simulink model "EnrouleurHG"  (R2024b)
settings: Solver=VariableStepAuto  StartTime=0.0  StopTime=.8  RelTol=1e-3
InitFcn:
  | run("parametres.m");
values from neighbouring files (symbols this model uses):
  fv = 0    [parametres.m]
  ISAT = 4    [parametres.m]
  Jm = 13.1/1000/10000    (= 1.31e-06)    [parametres.m]
  Kadapt = Kcapt/Rt    (= 52.1518917524)    [parametres.m]
  Kcapt = 8192/2/pi    (= 1303.79729381)    [parametres.m]
  Kcm = 25.5e-3    (= 0.0255)    [parametres.m]
  KCou_I = 900    [parametres.m]
  KCou_P = 2000    [parametres.m]
  KDSI = KPos_D*80/1000000    (= 0.0736)    [parametres.m]
  Kem = 1/(374 *2*pi/60)    (= 0.0255328785709)    [parametres.m]
  KPos_I = 270    [parametres.m]
  KPos_P = 215    [parametres.m]
  KPSI = KPos_P*10/1000    (= 2.15)    [parametres.m]
  Lm = 0.77e-3    (= 0.00077)    [parametres.m]
  r = 1/18    (= 0.0555555555556)    [parametres.m]
  Rm = 7.36    [parametres.m]
  Rt = 25    [parametres.m]
  Unom = 24    [parametres.m]
libraries: simulink x2
settings Model: Creator=xavier.pessoles2  LastModifiedBy=xpess

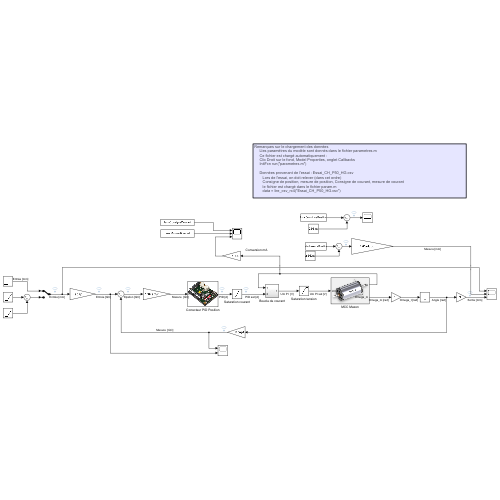
[thumbnail: Simulink's stored preview of the top-level diagram]
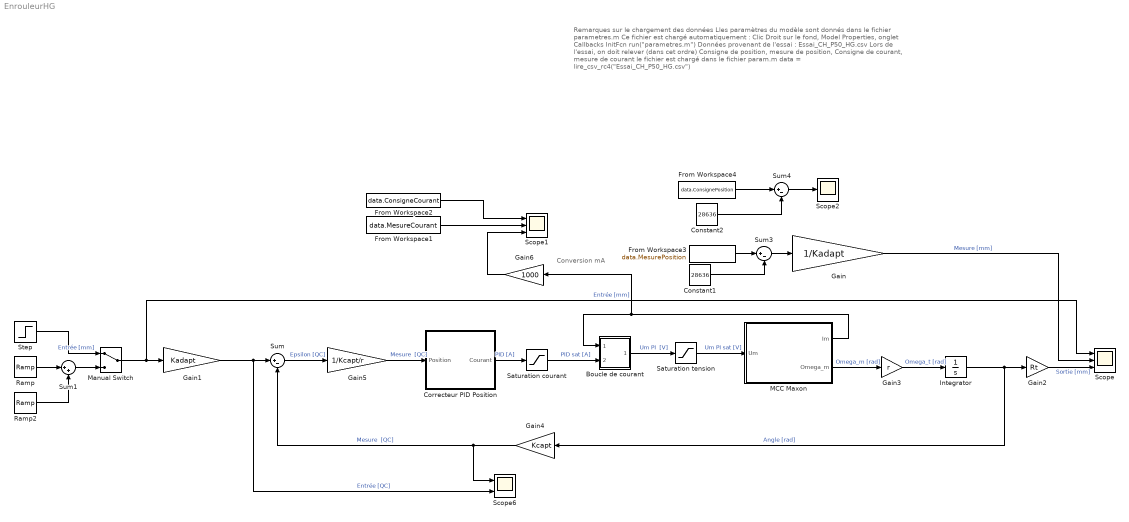
== system EnrouleurHG ==
  note: Conversion mA
  note: Remarques sur le chargement des données
      |      Lles paramètres du modèle sont donnés dans le fichier parametres.m
      |      Ce fichier est chargé automatiquement :
      |      Clic Droit sur le fond, Model Properties, onglet Callbacks
      |      InitFcn run("parametres.m")
      |
      |      Données provenant de l'essai : Essai_CH_P50_HG.csv
      |         Lors de l'essai, on doit relever (dans cet ordre)
      |         Consigne de position, mesure de position, Consigne de courant, mesure de courant
      |         le fichier est chargé dans le fichier param.m
      |         data = lire_csv_rc4("Essai_CH_P50_HG.csv")
  Boucle de courant : Subsystem
  Constant1 : Constant  Value=28636
  Constant2 : Constant  Value=28636
  Correcteur PID Position : Subsystem
      mask Display: image('EPOS.png');
  From Workspace1 : FromWorkspace  VariableName=data.MesureCourant  SampleTime=0.01
  From Workspace2 : FromWorkspace  VariableName=data.ConsigneCourant  SampleTime=0.01
  From Workspace3 : FromWorkspace  VariableName=data.MesurePosition  SampleTime=0.01
  From Workspace4 : FromWorkspace  VariableName=data.ConsignePosition  SampleTime=0.01
  Gain : Gain  Gain=1/Kadapt
  Gain1 : Gain  Gain=Kadapt
  Gain2 : Gain  Gain=Rt
  Gain3 : Gain  Gain=r
  Gain4 : Gain  Gain=Kcapt
  Gain5 : Gain  Gain=1/Kcapt/r
  Gain6 : Gain  Gain=1000
  Integrator : Integrator
  MCC Maxon : Subsystem
      mask Display: image('MCC.png');
  Manual Switch : ManualSwitch
  Ramp : simulink/Sources/Ramp  slope=378  start=0  InitialOutput=0
  Ramp2 : simulink/Sources/Ramp  slope=-378  start=1  InitialOutput=0
  Saturation courant : Saturate  UpperLimit=ISAT  LowerLimit=-ISAT
  Saturation tension : Saturate  UpperLimit=Unom  LowerLimit=-Unom
  Scope : Scope  NumInputPorts=3
  Scope1 : Scope  NumInputPorts=3
  Scope2 : Scope
  Scope6 : Scope  NumInputPorts=2
  Step : Step  Time=.08  After=50  SampleTime=0
  Sum : Sum  Inputs=|+-
  Sum1 : Sum  Inputs=|++
  Sum3 : Sum  Inputs=|+-
  Sum4 : Sum  Inputs=|+-
  wires:
  Gain3/1 -> Integrator/1  "Omega_t [rad]"
  MCC Maxon/2(Omega_m) -> Gain3/1  "Omega_m [rad]"
  Sum/1 -> Gain5/1  "Epsilon [QC]"
  MCC Maxon/1(Im) -> Gain6/1, Boucle de courant/1(In1)
  Correcteur PID Position/1(Courant) -> Saturation courant/1  "PID [A]"
  Boucle de courant/1(Out1) -> Saturation tension/1  "Um PI  [V]"
  Gain4/1 -> Scope6/1, Sum/2  "Mesure  [QC]"
  Gain1/1 -> Sum/1, Scope6/2  "Entrée [QC]"
  Gain2/1 -> Scope/3  "Sortie [mm]"
  Saturation tension/1 -> MCC Maxon/1(Um)  "Um PI sat [V]"
  Saturation courant/1 -> Boucle de courant/2(In2)  "PID sat [A]"
  Integrator/1 -> Gain2/1, Gain4/1  "Angle [rad]"
  Ramp/1 -> Sum1/1
  Ramp2/1 -> Sum1/2
  Sum1/1 -> Manual Switch/2
  Manual Switch/1 -> Gain1/1, Scope/1  "Entrée [mm]"
  Gain5/1 -> Correcteur PID Position/1(Position)  "Mesure  [QC]"
  Step/1 -> Manual Switch/1  "Entrée [mm]"
  From Workspace1/1 -> Scope1/2
  From Workspace2/1 -> Scope1/1
  From Workspace4/1 -> Sum4/1
  Gain/1 -> Scope/2  "Mesure [mm]"
  From Workspace3/1 -> Sum3/1
  Sum3/1 -> Gain/1
  Constant1/1 -> Sum3/2
  Constant2/1 -> Sum4/2
  Sum4/1 -> Scope2/1
  Gain6/1 -> Scope1/3

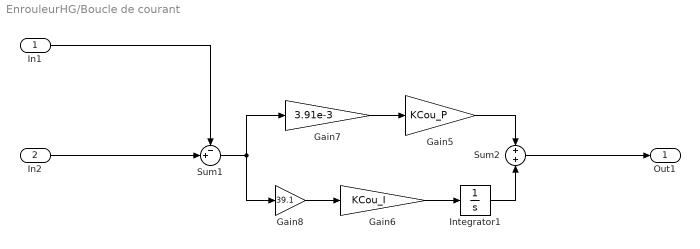
== system EnrouleurHG/Boucle de courant ==
  In1 : Inport
  In2 : Inport  Port=2
  Gain5 : Gain  Gain=KCou_P
  Gain6 : Gain  Gain=KCou_I
  Gain7 : Gain  Gain=3.91e-3
  Gain8 : Gain  Gain=39.1
  Integrator1 : Integrator
  Sum1 : Sum  Inputs=-+|
  Sum2 : Sum  Inputs=+|+
  Out1 : Outport
  wires:
  Sum1/1 -> Gain7/1, Gain8/1
  Gain5/1 -> Sum2/1
  Sum2/1 -> Out1/1
  Integrator1/1 -> Sum2/2
  Gain8/1 -> Gain6/1
  In1/1 -> Sum1/1
  Gain7/1 -> Gain5/1
  Gain6/1 -> Integrator1/1
  In2/1 -> Sum1/2

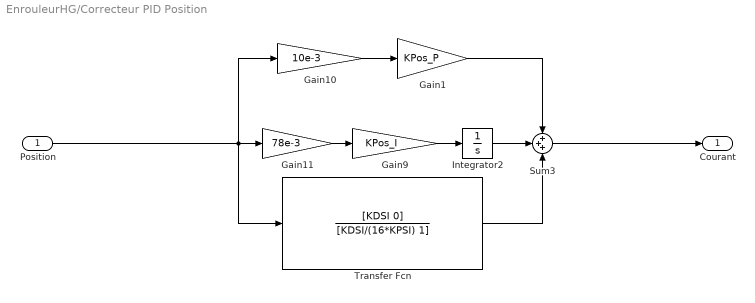
== system EnrouleurHG/Correcteur PID Position ==
  Position : Inport
  Gain1 : Gain  Gain=KPos_P
  Gain10 : Gain  Gain=10e-3
  Gain11 : Gain  Gain=78e-3
  Gain9 : Gain  Gain=KPos_I
  Integrator2 : Integrator
  Sum3 : Sum  Inputs=+++
  Transfer Fcn : TransferFcn  Numerator=[KDSI 0]  Denominator=[KDSI/(16*KPSI) 1]
  Courant : Outport
  wires:
  Gain1/1 -> Sum3/1
  Position/1 -> Gain10/1, Transfer Fcn/1, Gain11/1
  Gain9/1 -> Integrator2/1
  Sum3/1 -> Courant/1
  Integrator2/1 -> Sum3/2
  Gain10/1 -> Gain1/1
  Gain11/1 -> Gain9/1
  Transfer Fcn/1 -> Sum3/3

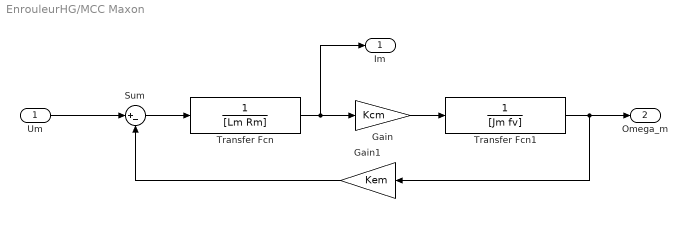
== system EnrouleurHG/MCC Maxon ==
  Um : Inport
  Gain : Gain  Gain=Kcm
  Gain1 : Gain  Gain=Kem
  Sum : Sum  Inputs=|+-
  Transfer Fcn : TransferFcn  Denominator=[Lm Rm]
  Transfer Fcn1 : TransferFcn  Denominator=[Jm fv]
  Im : Outport
  Omega_m : Outport  Port=2
  wires:
  Transfer Fcn/1 -> Im/1, Gain/1
  Transfer Fcn1/1 -> Omega_m/1, Gain1/1
  Gain/1 -> Transfer Fcn1/1
  Gain1/1 -> Sum/2
  Um/1 -> Sum/1
  Sum/1 -> Transfer Fcn/1
